simulink model "Conventional DTC"  (R2022a)
settings: Solver=ode1  StartTime=0.0  StopTime=Inf  FixedStep=Ts  RelTol=1e-3  EnableMultiTasking=on
PostLoadFcn:
  | , if any(exist('dsrtsu_mdlpostloadfcn', 'file') ~= 0), dsrtsu_mdlpostloadfcn('Execute', bdroot); end,
InitFcn:
  | , if any(exist('rtifpga_mdlclblib', 'file') ~= 0), rtifpga_mdlclblib('Init', bdroot); end,
undefined symbols (not defined in the file): P, Rs, Ts
libraries: rtilib1104 x15, rtitasklib x1
settings Model: DSRTSU_INTERNAL_RTI_VER=600  DSRTSU_INTERNAL_RTI_TYPE=rti1104  DSRTSU_INTERNAL_RTIFPGA=180  DSRTSU_INTERNAL_RTISTBM_VER=1.4.4  Creator=Admin  LastModifiedBy=acer
settings SolverCC: AlgebraicLoopSolver=TrustRegion
settings DataIOCC: LimitDataPoints=on  SaveFormat=Array  SignalLoggingSaveFormat=ModelDataLogs  ReturnWorkspaceOutputs=off
settings OptimizationCC: BlockReduction=off  ConditionallyExecuteInputs=off  OptimizeBlockIOStorage=off  BufferReuse=off  GlobalBufferReuse=off  ExpressionFolding=off  ExpressionDepthLimit=2147483647  LocalBlockOutputs=off  LifeSpan=inf
settings DebuggingCC: UnderspecifiedInitializationDetection=Classic  MergeDetectMultiDrivingBlocksExec=none  SolverPrmCheckMsg=warning  MultiTaskDSMMsg=warning  MultiTaskCondExecSysMsg=none  FcnCallInpInsideContextMsg=warning  UnconnectedInputMsg=warning  UnconnectedOutputMsg=warning  UnconnectedLineMsg=warning  StateNameClashWarn=warning  SFUnexpectedBacktrackingDiag=warning  SFNoUnconditionalDefaultTransitionDiag=warning  SFExecutionAtInitializationDiag=none  SFMachineParentedDataDiag=warning  ArithmeticOperatorsInVariantConditions=warning
settings HardwareCC: ProdBitPerPointer=32  ProdBitPerSizeT=32  ProdBitPerPtrDiffT=32  ProdLargestAtomicInteger=Integer  ProdEndianess=BigEndian  ProdWordSize=32  ProdHWDeviceType=Custom Processor->Custom  TargetIntDivRoundTo=Zero  TargetEndianess=BigEndian  TargetHWDeviceType=Custom Processor->Custom
settings ModelReferenceCC: PropagateSignalLabelsOutOfModel=off
settings SFSimCC: SimUseLocalCustomCode=off  MATLABDynamicMemAlloc=off  CustomCodeUndefinedFunction=UseInterfaceOnly
settings RTWCC: Description=dSPACE DS1104 Hardware Platform  SystemTargetFile=rti1104.tlc  MakeCommand=make_rti  TemplateMakefile=rti1104.tmf  RTWUseLocalCustomCode=off
settings CodeAppCC: StateflowObjectComments=on
settings STFCustomTargetCC: ParMdlRefBuildCompliant=on  GRTInterface=off  SystemTargetFile=rti1104.tlc
settings GRTTargetCC: TargetLangStandard=C89/C90 (ANSI)  CompOptLevelCompliant=off  ConcurrentExecutionCompliant=off  CombineOutputUpdateFcns=off  MatFileLogging=off  CPPClassGenCompliant=off  UseToolchainInfoCompliant=off  ExtModeMexFile=noextcomm
settings ConfigComp: CovMetricSettings=dw  CovSaveCumulativeToWorkspaceVar=on  CovSaveSingleToWorkspaceVar=on  CovExternalEMLEnable=off

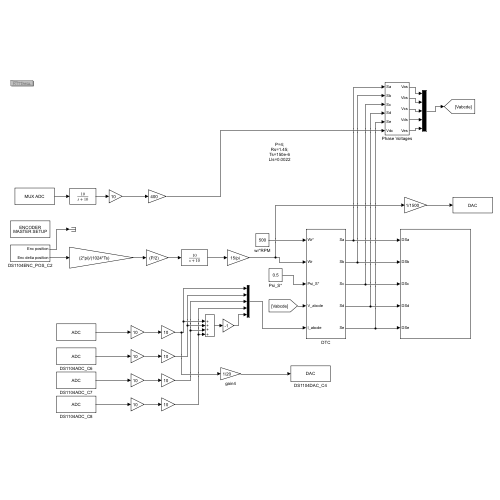
[thumbnail: Simulink's stored preview of the top-level diagram]
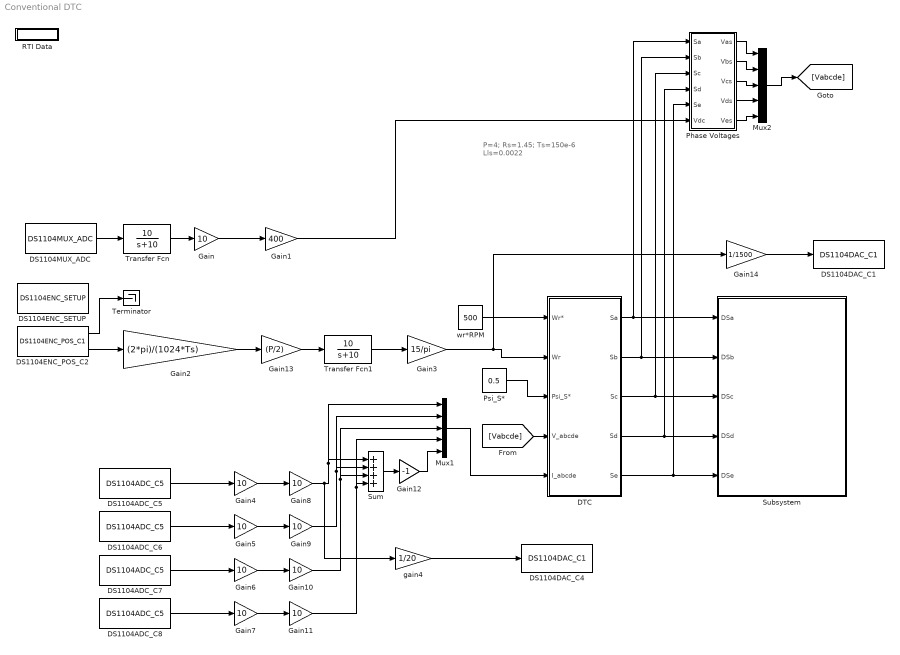
== system Conventional DTC ==
  note: P=4;
      | Rs=1.45;
      | Ts=150e-6
      | Lls=0.0022
  DS1104ADC_C5 : rtilib1104/DS1104 MASTER PPC/DS1104ADC_C5  ChannelNo=5  TriggerMode=0  Reserved1=[]  Reserved2=[]  Reserved3=[]  Reserved4=[]  DialogFcn=gui1104adc  UnitName={ 'DS1104ADC_C' }  UnitValues={ 5 }  DSProperties=struct('RTI',struct('Version',uint32(1),'BlockType',struct('isSLSource',uint8(1),'isSLSink',uint8(0),'isHWSource',uint8(1),'isHWSink',uint8(0),'isSetup',uint8(0),'isInline',uint8(1),'isNonInline',uint8(0),'isInterrupt',uint8(0),'isChannelwise',uint8(1)),'IOBoardType','DS1104MASTER','UnitType','ADC','Identifier','ADC','DialogType','ML','BlockSet','NONE','SlaveProcessor','NONE'))
      settings: SourceProductName=dSPACE RTI1104
  DS1104ADC_C6 : rtilib1104/DS1104 MASTER PPC/DS1104ADC_C5  ChannelNo=6  TriggerMode=0  Reserved1=[]  Reserved2=[]  Reserved3=[]  Reserved4=[]  DialogFcn=gui1104adc  UnitName={ 'DS1104ADC_C' }  UnitValues={ 6 }  DSProperties=struct('RTI',struct('Version',uint32(1),'BlockType',struct('isSLSource',uint8(1),'isSLSink',uint8(0),'isHWSource',uint8(1),'isHWSink',uint8(0),'isSetup',uint8(0),'isInline',uint8(1),'isNonInline',uint8(0),'isInterrupt',uint8(0),'isChannelwise',uint8(1)),'IOBoardType','DS1104MASTER','UnitType','ADC','Identifier','ADC','DialogType','ML','BlockSet','NONE','SlaveProcessor','NONE'))
      settings: SourceProductName=dSPACE RTI1104
  DS1104ADC_C7 : rtilib1104/DS1104 MASTER PPC/DS1104ADC_C5  ChannelNo=7  TriggerMode=0  Reserved1=[]  Reserved2=[]  Reserved3=[]  Reserved4=[]  DialogFcn=gui1104adc  UnitName={ 'DS1104ADC_C' }  UnitValues={ 7 }  DSProperties=struct('RTI',struct('Version',uint32(1),'BlockType',struct('isSLSource',uint8(1),'isSLSink',uint8(0),'isHWSource',uint8(1),'isHWSink',uint8(0),'isSetup',uint8(0),'isInline',uint8(1),'isNonInline',uint8(0),'isInterrupt',uint8(0),'isChannelwise',uint8(1)),'IOBoardType','DS1104MASTER','UnitType','ADC','Identifier','ADC','DialogType','ML','BlockSet','NONE','SlaveProcessor','NONE'))
      settings: SourceProductName=dSPACE RTI1104
  DS1104ADC_C8 : rtilib1104/DS1104 MASTER PPC/DS1104ADC_C5  ChannelNo=8  TriggerMode=0  Reserved1=[]  Reserved2=[]  Reserved3=[]  Reserved4=[]  DialogFcn=gui1104adc  UnitName={ 'DS1104ADC_C' }  UnitValues={ 8 }  DSProperties=struct('RTI',struct('Version',uint32(1),'BlockType',struct('isSLSource',uint8(1),'isSLSink',uint8(0),'isHWSource',uint8(1),'isHWSink',uint8(0),'isSetup',uint8(0),'isInline',uint8(1),'isNonInline',uint8(0),'isInterrupt',uint8(0),'isChannelwise',uint8(1)),'IOBoardType','DS1104MASTER','UnitType','ADC','Identifier','ADC','DialogType','ML','BlockSet','NONE','SlaveProcessor','NONE'))
      settings: SourceProductName=dSPACE RTI1104
  DS1104DAC_C1 : rtilib1104/DS1104 MASTER PPC/DS1104DAC_C1  ChannelNo=1  InitValue=0  TermMode=0  TermValue=0  Reserved1=[]  Reserved2=[]  Reserved3=[]  Reserved4=[]  DialogFcn=gui1104dac  UnitName={ 'DS1104DAC_C'}  UnitValues={ 1 }  DSProperties=struct('RTI',struct('Version',uint32(1),'BlockType',struct('isSLSource',uint8(0),'isSLSink',uint8(1),'isHWSource',uint8(0),'isHWSink',uint8(1),'isSetup',uint8(0),'isInline',uint8(1),'isNonInline',uint8(0),'isInterrupt',uint8(0),'isChannelwise',uint8(1)),'IOBoardType','DS1104MASTER','UnitType','DAC','Identifier','DAC','DialogType','ML','BlockSet','NONE','SlaveProcessor','NONE'))
      settings: SourceProductName=dSPACE RTI1104
  DS1104DAC_C4 : rtilib1104/DS1104 MASTER PPC/DS1104DAC_C1  ChannelNo=4  InitValue=0  TermMode=0  TermValue=0  Reserved1=[]  Reserved2=[]  Reserved3=[]  Reserved4=[]  DialogFcn=gui1104dac  UnitName={ 'DS1104DAC_C'}  UnitValues={4}  DSProperties=struct('RTI',struct('Version',uint32(1),'BlockType',struct('isSLSource',uint8(0),'isSLSink',uint8(1),'isHWSource',uint8(0),'isHWSink',uint8(1),'isSetup',uint8(0),'isInline',uint8(1),'isNonInline',uint8(0),'isInterrupt',uint8(0),'isChannelwise',uint8(1)),'IOBoardType','DS1104MASTER','UnitType','DAC','Identifier','DAC','DialogType','ML','BlockSet','NONE','SlaveProcessor','NONE'))
      settings: SourceProductName=dSPACE RTI1104
  DS1104ENC_POS_C2 : rtilib1104/DS1104 MASTER PPC/DS1104ENC_POS_C1  ChannelNo=2  PosValue=0  Reserved1=[]  Reserved2=[]  Reserved3=[]  Reserved4=[]  DialogFcn=gui1104enc_pos  UnitName={'DS1104ENC_POS_C'}  UnitValues={ 2 }  DSProperties=struct('RTI',struct('Version',uint32(1),'BlockType',struct('isSLSource',uint8(1),'isSLSink',uint8(0),'isHWSource',uint8(1),'isHWSink',uint8(0),'isSetup',uint8(0),'isInline',uint8(1),'isNonInline',uint8(0),'isInterrupt',uint8(0),'isChannelwise',uint8(1)),'IOBoardType','DS1104MASTER','UnitType','ENC','Identifier','ENCPOSCH','DialogType','ML','BlockSet','NONE','SlaveProcessor','NONE'))
      settings: SourceProductName=dSPACE RTI1104
  DS1104ENC_SETUP : rtilib1104/DS1104 MASTER PPC/DS1104ENC_SETUP  Reserved1=[]  Reserved2=[]  Reserved3=[]  Reserved4=[]  DialogFcn=gui1104enc_setup  UnitName={'DS1104ENC_SETUP'}  UnitValues={ [] }  DSProperties=struct('RTI',struct('Version',uint32(1),'BlockType',struct('isSLSource',uint8(0),'isSLSink',uint8(0),'isHWSource',uint8(0),'isHWSink',uint8(0),'isSetup',uint8(0),'isInline',uint8(1),'isNonInline',uint8(0),'isInterrupt',uint8(0),'isChannelwise',uint8(0)),'IOBoardType','DS1104MASTER','UnitType','ENC','Identifier','ENCSETUP','DialogType','ML','BlockSet','NONE','SlaveProcessor','NONE'))
      settings: SourceProductName=dSPACE RTI1104  SignalType=[0 0]
  DS1104MUX_ADC : rtilib1104/DS1104 MASTER PPC/DS1104MUX_ADC  ChannelNos=1  TriggerMode=0  Reserved1=[]  Reserved2=[]  Reserved3=[]  Reserved4=[]  DialogFcn=gui1104mux_adc  UnitName={ 'DS1104MUX_ADC' }  UnitValues={ [] }  DSProperties=struct('RTI',struct('Version',uint32(1),'BlockType',struct('isSLSource',uint8(1),'isSLSink',uint8(0),'isHWSource',uint8(1),'isHWSink',uint8(0),'isSetup',uint8(0),'isInline',uint8(1),'isNonInline',uint8(0),'isInterrupt',uint8(0),'isChannelwise',uint8(0)),'IOBoardType','DS1104MASTER','UnitType','ADC','Identifier','ADCMUX','DialogType','ML','BlockSet','NONE','SlaveProcessor','NONE'))
      settings: SourceProductName=dSPACE RTI1104
  DTC : Subsystem
  Gain{,4..11} (9 alike) : Gain  Gain=10
  Gain1 : Gain  Gain=400
  Gain12 : Gain  Gain=-1
  Gain13 : Gain  Gain=(P/2)
  Gain14 : Gain  Gain=1/1500
  Gain2 : Gain  Gain=(2*pi)/(1024*Ts)
  Gain3 : Gain  Gain=15/pi
  Mux1 : Mux  Inputs=5
  Mux2 : Mux  Inputs=5
  Phase Voltages : Subsystem
  Psi_S* : Constant  Value=0.5
  RTI Data : Subsystem  Tag=struct('RTIDataServer',struct('RTIDataServerVs','2','RTIModelDescription','struct(''main'',''Modified_DTC_PWMnD'',''sub'','''',''isMp'',0)'))  LoadFcn="if exist('rtidc'), try,  rtidc('DataHostBlockClbLoad', gcbh); catch, disp(['Warning: ''LoadFcn'' for RTI Data block failed: ' lasterr]); end, end,"  mask(RTI_DATA_HOST){}
      mask help:
      | RTI Data Block.
      | This block is used by RTI to store internal model-dependent data.
      | Please keep this block on the root level of the model. Deleting this block will result in data loss.
      |
      | NEVER DELETE OR COPY THIS BLOCK!
      settings: CopyFcn="if exist('rtidc'), try,  rtidc('DataHostBlockClbCopy', gcbh); catch, disp(['Warning: ''CopyFcn'' for RTI Data block failed: ' lasterr]); end, end,"  DeleteFcn="if exist('rtidc'), try,  rtidc('DataHostBlockClbDelete', gcbh); catch, disp(['Warning: ''DeleteFcn'' for RTI Data block failed: ' lasterr]); end, end,"  ModelCloseFcn="if exist('rtidc'), try,  rtidc('DataHostBlockClbModelClose', gcbh); catch, disp(['Warning: ''ModelCloseFcn'' for RTI Data block failed: ' lasterr]); end, end,"  PreSaveFcn="if exist('rtidc'), try,  rtidc('DataHostBlockClbPreSave', gcbh); catch, disp(['Warning: ''PreSaveFcn'' for RTI Data block failed: ' lasterr]); end, end,"  PostSaveFcn="if exist('rtidc'), try,  rtidc('DataHostBlockClbPostSave', gcbh); catch, disp(['Warning: ''PostSaveFcn'' for RTI Data block failed: ' lasterr]); end, end,"  NameChangeFcn="if exist('rtidc'), try,  rtidc('DataHostBlockClbNameChange', gcbh); catch, disp(['Warning: ''NameChangeFcn'' for RTI Data block failed: ' lasterr]); end, end,"
      mask Help:
      | RTI Data Block.
      | This block is used by RTI to store internal model-dependent data.
      | Please keep this block on the root level of the model. Deleting this block will result in data loss.
      | 
      | NEVER DELETE OR COPY THIS BLOCK!
      mask Display:
      | text(0.5, 0.5, 'RTI Data', 'HorizontalAlignment', 'center');
      | plot([1 0]);
  Subsystem : Subsystem
  Sum : Sum  Inputs=|++++
  Terminator : Terminator
  Transfer Fcn : TransferFcn  Numerator=[10]  Denominator=[1 10]
  Transfer Fcn1 : TransferFcn  Numerator=[10]  Denominator=[1 10]
  gain4 : Gain  Gain=1/20  SaturateOnIntegerOverflow=on  OutDataTypeStr=Inherit: Same as input  ParamDataTypeStr=Inherit: Same as input
  wr*RPM : Constant  Value=500
  wires:
  wr*RPM/1 -> DTC/1(Wr*)
  [Vabcde] -> DTC/4(V_abcde)
  Psi_S*/1 -> DTC/3(Psi_S*)
  Gain/1 -> Gain1/1
  Transfer Fcn/1 -> Gain/1
  Gain4/1 -> Gain8/1
  Gain5/1 -> Gain9/1
  Gain6/1 -> Gain10/1
  Gain7/1 -> Gain11/1
  Gain9/1 -> Mux1/2, Sum/2
  Gain10/1 -> Mux1/3, Sum/3
  Gain11/1 -> Mux1/4, Sum/4
  Mux1/1 -> DTC/5(I_abcde)
  Phase Voltages/1(Vas) -> Mux2/1
  Phase Voltages/2(Vbs) -> Mux2/2
  Phase Voltages/3(Vcs) -> Mux2/3
  Phase Voltages/4(Vds) -> Mux2/4
  Phase Voltages/5(Ves) -> Mux2/5
  Mux2/1 -> [Vabcde]
  DTC/1(Sa) -> Phase Voltages/1(Sa), Subsystem/1(DSa)
  DTC/2(Sb) -> Subsystem/2(DSb), Phase Voltages/2(Sb)
  DTC/3(Sc) -> Subsystem/3(DSc), Phase Voltages/3(Sc)
  DTC/4(Sd) -> Subsystem/4(DSd), Phase Voltages/4(Sd)
  DTC/5(Se) -> Subsystem/5(DSe), Phase Voltages/5(Se)
  Sum/1 -> Gain12/1
  Gain12/1 -> Mux1/5
  DS1104ADC_C5/1 -> Gain4/1
  DS1104ADC_C6/1 -> Gain5/1
  DS1104ADC_C7/1 -> Gain6/1
  DS1104ADC_C8/1 -> Gain7/1
  Transfer Fcn1/1 -> Gain3/1
  DS1104MUX_ADC/1 -> Transfer Fcn/1
  DS1104ENC_POS_C2/2 -> Gain2/1
  Gain2/1 -> Gain13/1
  Gain13/1 -> Transfer Fcn1/1
  DS1104ENC_POS_C2/1 -> Terminator/1
  Gain1/1 -> Phase Voltages/6(Vdc)
  Gain14/1 -> DS1104DAC_C1/1
  Gain3/1 -> Gain14/1, DTC/2(Wr)
  Gain8/1 -> gain4/1, Mux1/1, Sum/1
  gain4/1 -> DS1104DAC_C4/1

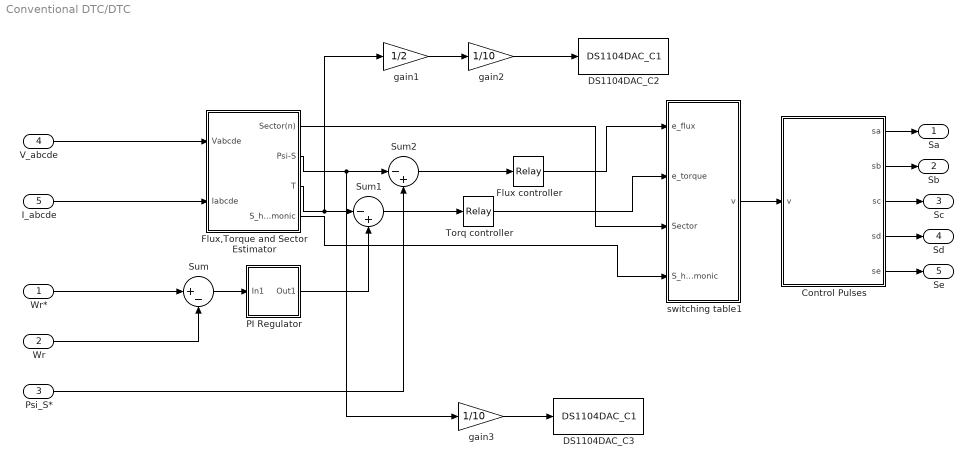
== system Conventional DTC/DTC ==
  Wr* : Inport
  Wr : Inport  Port=2
  Psi_S* : Inport  Port=3
  V_abcde : Inport  Port=4
  I_abcde : Inport  Port=5
  Control Pulses : MATLAB Function  TreatAsAtomicUnit=on
  DS1104DAC_C2 : rtilib1104/DS1104 MASTER PPC/DS1104DAC_C1  ChannelNo=2  InitValue=0  TermMode=0  TermValue=0  Reserved1=[]  Reserved2=[]  Reserved3=[]  Reserved4=[]  DialogFcn=gui1104dac  UnitName={ 'DS1104DAC_C'}  UnitValues={ 2 }  DSProperties=struct('RTI',struct('Version',uint32(1),'BlockType',struct('isSLSource',uint8(0),'isSLSink',uint8(1),'isHWSource',uint8(0),'isHWSink',uint8(1),'isSetup',uint8(0),'isInline',uint8(1),'isNonInline',uint8(0),'isInterrupt',uint8(0),'isChannelwise',uint8(1)),'IOBoardType','DS1104MASTER','UnitType','DAC','Identifier','DAC','DialogType','ML','BlockSet','NONE','SlaveProcessor','NONE'))
      settings: SourceProductName=dSPACE RTI1104
  DS1104DAC_C3 : rtilib1104/DS1104 MASTER PPC/DS1104DAC_C1  ChannelNo=3  InitValue=0  TermMode=0  TermValue=0  Reserved1=[]  Reserved2=[]  Reserved3=[]  Reserved4=[]  DialogFcn=gui1104dac  UnitName={ 'DS1104DAC_C'}  UnitValues={ 3 }  DSProperties=struct('RTI',struct('Version',uint32(1),'BlockType',struct('isSLSource',uint8(0),'isSLSink',uint8(1),'isHWSource',uint8(0),'isHWSink',uint8(1),'isSetup',uint8(0),'isInline',uint8(1),'isNonInline',uint8(0),'isInterrupt',uint8(0),'isChannelwise',uint8(1)),'IOBoardType','DS1104MASTER','UnitType','DAC','Identifier','DAC','DialogType','ML','BlockSet','NONE','SlaveProcessor','NONE'))
      settings: SourceProductName=dSPACE RTI1104
  Flux controller : Relay  OnSwitchValue=0.01  OffSwitchValue=-0.01  OffOutputValue=-1
  Flux,Torque and Sector Estimator : Subsystem
  PI Regulator : Subsystem
  Sum : Sum  Inputs=|+-
  Sum1 : Sum  Inputs=|-+
  Sum2 : Sum  Inputs=|-+
  Torq controller : Relay  OnSwitchValue=0.5  OffSwitchValue=-0.5  OffOutputValue=-1
  gain1 : Gain  Gain=1/2  SaturateOnIntegerOverflow=on  OutDataTypeStr=Inherit: Same as input  ParamDataTypeStr=Inherit: Same as input
  gain2 : Gain  Gain=1/10  SaturateOnIntegerOverflow=on  OutDataTypeStr=Inherit: Same as input  ParamDataTypeStr=Inherit: Same as input
  gain3 : Gain  Gain=1/10  SaturateOnIntegerOverflow=on  OutDataTypeStr=Inherit: Same as input  ParamDataTypeStr=Inherit: Same as input
  switching table1 : Subsystem
  Sa : Outport
  Sb : Outport  Port=2
  Sc : Outport  Port=3
  Sd : Outport  Port=4
  Se : Outport  Port=5
  wires:
  PI Regulator/1(Out1) -> Sum1/2
  Flux controller/1 -> switching table1/1(e_flux)
  Sum2/1 -> Flux controller/1
  Wr/1 -> Sum/2
  Psi_S*/1 -> Sum2/2
  Sum/1 -> PI Regulator/1(In1)
  V_abcde/1 -> Flux,Torque and Sector Estimator/1(Vabcde)
  switching table1/1(v) -> Control Pulses/1(v)
  Control Pulses/1(sa) -> Sa/1
  Control Pulses/2(sb) -> Sb/1
  Control Pulses/3(sc) -> Sc/1
  Control Pulses/4(sd) -> Sd/1
  Control Pulses/5(se) -> Se/1
  I_abcde/1 -> Flux,Torque and Sector Estimator/2(Iabcde)
  Sum1/1 -> Torq controller/1
  Torq controller/1 -> switching table1/2(e_torque)
  Flux,Torque and Sector Estimator/4(S_harmonic) -> switching table1/4(S_harmonic)
  Wr*/1 -> Sum/1
  gain1/1 -> gain2/1
  gain2/1 -> DS1104DAC_C2/1
  Flux,Torque and Sector Estimator/3(T) -> gain1/1, Sum1/1
  gain3/1 -> DS1104DAC_C3/1
  Flux,Torque and Sector Estimator/2(Psi-S) -> gain3/1, Sum2/1
  Flux,Torque and Sector Estimator/1(Sector(n)) -> switching table1/3(Sector)

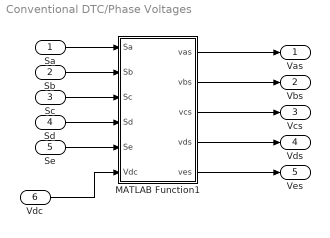
== system Conventional DTC/Phase Voltages ==
  Sa : Inport
  Sb : Inport  Port=2
  Sc : Inport  Port=3
  Sd : Inport  Port=4
  Se : Inport  Port=5
  Vdc : Inport  Port=6
  MATLAB Function1 : MATLAB Function  TreatAsAtomicUnit=on
  Vas : Outport
  Vbs : Outport  Port=2
  Vcs : Outport  Port=3
  Vds : Outport  Port=4
  Ves : Outport  Port=5
  wires:
  Sa/1 -> MATLAB Function1/1(Sa)
  Sb/1 -> MATLAB Function1/2(Sb)
  Sc/1 -> MATLAB Function1/3(Sc)
  Sd/1 -> MATLAB Function1/4(Sd)
  Se/1 -> MATLAB Function1/5(Se)
  MATLAB Function1/1(vas) -> Vas/1
  MATLAB Function1/4(vds) -> Vds/1
  MATLAB Function1/5(ves) -> Ves/1
  Vdc/1 -> MATLAB Function1/6(Vdc)
  MATLAB Function1/2(vbs) -> Vbs/1
  MATLAB Function1/3(vcs) -> Vcs/1

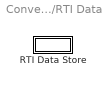
== system Conventional DTC/RTI Data ==
  RTI Data Store : Subsystem  Tag="struct('public',struct('sub',struct('name',{{'Modified_DTC_PWMnD'}},'data',{{struct('TH',struct('thTaskInfo',struct('taskType',{'TIMER','HWINT','TMRINT','SWINT','GLINT'},'tasksNumOf',{1,0,0,0,0},'srcIds',{{'PWMINT'},{},{},{},{}},'taskNames',{{['Timer Task 1']},{},{},{},{}})),'th_tc',struct('dataType','TASK','taskGroupId','','taskGroupList',{{}},'taskSchedulingPolicy','FCFS','taskType','TIMER','blkh','Modified_DTC_PWMnD/Subsystem/DS1104SLAVE_PWMINT1','srcId','PWMINT','srcSgnName',['SLAVE-PWM-Interrupt with variable alignment'],'srcCpuName','','taskName',['Timer Task 1  [0.00015] s'],'taskNameDisplayExt','','smplTime',0.00015,'smplTimeOffs',0,'hasFixedPriority',0,'priority',1,'hasFixedOvc',0,'ovcType',1,'ovcMax',1),'tc_th',struct('dataType','TASK','taskGroupId','','taskGroupList',{{}},'taskSchedulingPolicy','FCFS','taskType','TIMER','blkh','Modified_DTC_PWMnD/Subsystem/DS1104SLAVE_PWMINT1','srcId','PWMINT','srcSgnName',['SLAVE-PWM-Interrupt with variable alignment'],'srcCpuName','','taskName',['Timer Task 1  [0.00015] s'],'taskNameDisplayExt','','smplTime',0.00015,'smplTimeOffs',0,'hasFixedPriority',0,'priority',1,'hasFixedOvc',0,'ovcType',1,'ovcMax',1))}})),'private',struct('version',struct('dsVer',uint32(2)),'access',struct('modified',['16-Jul-2024 11:25:11'],'type','Model','isPerm',1)))"  mask(RTI_DATA_STORE){}
      mask help:
      | RTI Data Store Block. This block is used by RTI to store internal model dependent data. Deleting this block will result in data loss.
      |
      | NEVER DELETE, COPY, OR MODIFY THIS BLOCK!
      mask Help:
      | RTI Data Store Block. This block is used by RTI to store internal model dependent data. Deleting this block will result in data loss.
      | 
      | NEVER DELETE, COPY, OR MODIFY THIS BLOCK!
      mask Display: text(0.5, 0.5, ' ', 'HorizontalAlignment', 'center');

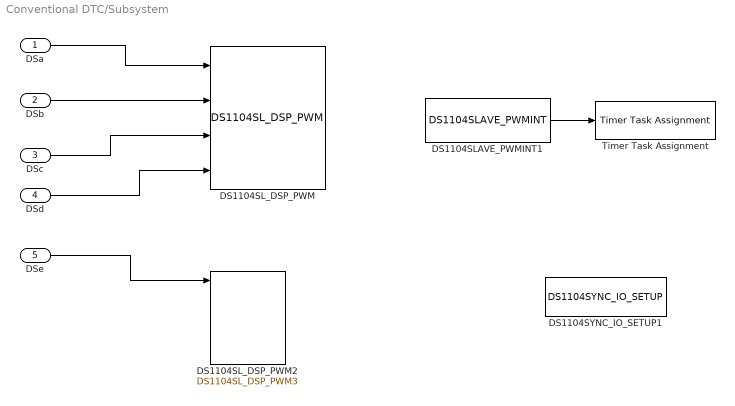
== system Conventional DTC/Subsystem ==
  DSa : Inport
  DSb : Inport  Port=2
  DSc : Inport  Port=3
  DSd : Inport  Port=4
  DSe : Inport  Port=5
  DS1104SLAVE_PWMINT1 : rtilib1104/DS1104 SLAVE DSP/DS1104SLAVE_PWMINT  Parameters=[]  TDef=[]  BoardIntNo=[]  InterruptName=[]  Delay=[]  DialogFcn=[]  Reserved1=[]  Reserved2=[]  Reserved3=[]  Reserved4=[]  Revision=[]  UnitName=[]  UnitValues=[]  DSProperties=struct('RTI',struct('Version',uint32(530),'IOBoardType','DS1104SLAVE','SlaveProcessor','F240','UnitType','HWINT','Identifier','PWMINT','BlockType',struct('isSLSource',uint8(1),'isSLSink',uint8(0),'isHWSource',uint8(1),'isHWSink',uint8(0),'isSetup',uint8(0),'isInline',uint8(1),'isNonInline',uint8(0),'isInterrupt',uint8(1),'isChannelwise',uint8(0)),'DialogType','ML','BlockSet','NONE','RelationId',struct('TH',struct('BlockId','HWINT'))))  RTIBlockInterface=struct('BlockName',struct('Token',{{'DS1104SLAVE_PWMINT'}}),'BlockDisplay',{{['DS1104SLAVE Board \nPWM-Interrupt'],'center'}},'DialogFcn','rti110xhwintgui','OutputPortsActive',1,'OutputPortsWidth',int32(1),'FunctionCall',uint32(0),'OutputPortsName',{{[' ']}},'IconTransparency','on','InitLevel',3,'Options',{{'SS_OPTION_FORCE_NONINLINED_FCNCALL','SS_OPTION_ASYNCHRONOUS_INTERRUPT'}},'OutputPortsDataType',{{'SS_FCN_CALL'}})  RTIBlockParameters=struct('ThIntNo',{{10,'OFF',[]}},'IntDelay',{{0.01,'ON',[1e-6 1]}},'ThSrcSgnName',{{['SLAVE-PWM-Interrupt with variable alignment'],'OFF',[]}},'TLCFileName',{{'rti1104slave_pwm_interrupt','OFF',[]}},'ThBlk',{{['struct(''blkh'',''Modified_DTC_PWMnD/Subsystem/DS1104SLAVE_PWMINT1'',''srcId'',''PWMINT'',''srcSgnId'',''PWMINT'',''intervalTmrBlockId'',[],''srcSgnName'',[''SLAVE-PWM-Interrupt with variable alignment''],''srcCpuId'','''',''isSrcCpu'',1,''isTargetCpu'',1,''srcOnMasterCpu'',1,''boardType'','''',''boardTypeNo'','''',''boardNo'',1,''intNo'',0,''subIntNo'',-1,''period'',0,''entryPoint'',''rti_PWMINT'',''blockName'',''DS1104SLAVE_PWMINT1'',''taskNameDisplayExt'','''',''taskType'',''HWINT'',''groupId'',''PWMINT'',''hookFcn'',''NULL'',''isTimerTaskSrc'',1,''service'','''',''mpBlkId'','''',''taskPriorityPreConfig'',''none'',''taskPriority'',-1,''taskSortWeighting'',[],''taskSchedulingPolicy'',''FCFS'',''taskOvrPreConfig'',''none'',''taskOvrStrategy'',1,''taskOvrQueueSize'',1,''taskVisibility'',''on'',''taskGroupId'','''',''taskGroupDisplayOrder'',[],''serviceDynamicGen'',0,''disableCodeGen'',0,''boardBase'',''0'',''noBoardBase'','''')'],'OFF',[]}},'PHSBoardBaseId',{{'DSXXXX','OFF',[]}})  RTISFcnParameters=struct('IntDelay','double','ThBlk','struct','ThIntNo','int32','TLCFileName','char','PHSBoardBaseId','char')  RTIBlockParaDefault=struct('ThIntNo',10,'IntDelay',2^-1,'ThSrcSgnName',['SLAVE-PWM-Interrupt with none delay'],'TLCFileName','rti1104slave_pwm_interrupt','ThBlk',['struct(''srcSgnId'', '''')'],'PHSBoardBaseId','DSXXXX')
      settings: SourceProductName=dSPACE RTI1104
  DS1104SL_DSP_PWM : rtilib1104/DS1104 SLAVE DSP/DS1104SL_DSP_PWM  Parameters=[]  TDef=[]  BoardType=[]  PwmMode=[]  Frequency=[]  InitValue=[]  TermMode=[]  TermValue=[]  Polarity=[]  DialogFcn=[]  Reserved1=[]  Reserved2=[]  Reserved3=[]  Reserved4=[]  Revision=[]  UnitName=[]  UnitValues=[]  DSProperties=struct('RTI',struct('Version',uint32(2),'BlockType',struct('isSLSource',uint8(0),'isSLSink',uint8(1),'isHWSource',uint8(0),'isHWSink',uint8(1),'isSetup',uint8(0),'isInline',uint8(1),'isNonInline',uint8(0),'isInterrupt',uint8(0),'isChannelwise',uint8(0)),'IOBoardType','DS1104SLAVE','UnitType','PWM','Identifier','PWM','DialogType','ML','BlockSet','NONE','SlaveProcessor','F240'))  RTIBlockInterface=struct('InputPortsActive',[1 1 1 1],'InputPortsWidth',int32([1 1 1 1]),'InputPortsName',{{['PWM Channel 1'],['PWM Channel 2'],['PWM Channel 3'],['PWM Channel 4']}},'IWork',{{{'',uint32(4)}}},'DialogFcn','rti1104slavepwmgui','InitLevel',1,'BlockDisplay',{{'','auto'}},'IconTransparency','on','MultiSFcn',4,'BlockName',struct('Token',{{'DS1104SL_DSP_PWM'}}))  RTIBlockParameters=struct('PWMSymmetryMode',{{1,'OFF',[]}},'PWMFrequency',{{'1/Ts','OFF',[]}},'PWMPolarityMode',{{[1 1 1 1 1],'OFF',[]}},'ChannelNo',{{[1 2 3 4],'OFF',[]}},'SuspendModeInit',{{[1 1 1 1 1],'OFF',[]}},'TTLModeInit',{{[2 2 2 2 2],'OFF',[]}},'DutyCycleInitValueCh1',{{'0.5','OFF',[]}},'DutyCycleInitValueCh2',{{'0.5','OFF',[]}},'DutyCycleInitValueCh3',{{'0.5','OFF',[]}},'DutyCycleInitValueCh4',{{'0.5','OFF',[]}},'DutyCycleInitValueCh5',{{'0.5','OFF',[]}},'EnablePWMStop',{{[0 0 0 0 0],'OFF',[]}},'SuspendModeTerm',{{[0 1 1 1 1],'OFF',[]}},'TTLModeTerm',{{[2 2 2 2 2],'OFF',[]}},'DutyCycleTermValueCh1',{{'0.5','OFF',[]}},'DutyCycleTermValueCh2',{{'0.5','OFF',[]}},'DutyCycleTermValueCh3',{{'0.5','OFF',[]}},'DutyCycleTermValueCh4',{{'0.5','OFF',[]}},'DutyCycleTermValueCh5',{{'0.5','OFF',[]}},'TLCFileName',{{'rti1104pwm','OFF',[]}})  RTISFcnParameters=struct('PWMSymmetryMode','double','PWMFrequency','double','PWMPolarityMode','double','ChannelNo','double','SuspendModeInit','double','TTLModeInit','double','DutyCycleInitValueCh1','double','DutyCycleInitValueCh2','double','DutyCycleInitValueCh3','double','DutyCycleInitValueCh4','double','EnablePWMStop','double','SuspendModeTerm','double','TTLModeTerm','double','DutyCycleTermValueCh1','double','DutyCycleTermValueCh2','double','DutyCycleTermValueCh3','double','DutyCycleTermValueCh4','double','TLCFileName','char')  RTIBlockParaDefault=struct('PWMSymmetryMode',1,'PWMFrequency',100,'PWMPolarityMode',[1 1 1 1 1],'ChannelNo',[1 2 3 4],'SuspendModeInit',[1 1 1 1 1],'TTLModeInit',[2 2 2 2 2],'DutyCycleInitValueCh1',2^-1,'DutyCycleInitValueCh2',2^-1,'DutyCycleInitValueCh3',2^-1,'DutyCycleInitValueCh4',2^-1,'DutyCycleInitValueCh5',2^-1,'EnablePWMStop',[1 1 1 1 0],'SuspendModeTerm',[1 1 1 1 1],'TTLModeTerm',[2 2 2 2 2],'DutyCycleTermValueCh1',2^-1,'DutyCycleTermValueCh2',2^-1,'DutyCycleTermValueCh3',2^-1,'DutyCycleTermValueCh4',2^-1,'DutyCycleTermValueCh5',2^-1,'TLCFileName','rti1104pwm')
      settings: SourceProductName=dSPACE RTI1104
  DS1104SL_DSP_PWM2 : rtilib1104/DS1104 SLAVE DSP/DS1104SL_DSP_PWM3  Parameters=[]  TDef=[]  BoardType=[]  PwmMode=[]  Frequency=[]  DeadBand=[]  InitValue=[]  TermMode=[]  TermValue=[]  IntDelay=[]  DialogFcn=[]  Reserved1=[]  Reserved2=[]  Reserved3=[]  Reserved4=[]  Revision=[]  UnitName=[]  UnitValues=[]  DSProperties=struct('RTI',struct('Version',uint32(2),'BlockType',struct('isSLSource',uint8(0),'isSLSink',uint8(1),'isHWSource',uint8(0),'isHWSink',uint8(1),'isSetup',uint8(0),'isInline',uint8(1),'isNonInline',uint8(0),'isInterrupt',uint8(0),'isChannelwise',uint8(0)),'IOBoardType','DS1104SLAVE','UnitType','PWM','Identifier','PWM3','DialogType','ML','BlockSet','NONE','SlaveProcessor','F240'))  RTIBlockInterface=struct('InputPortsActive',[1 1 1 1],'InputPortsWidth',int32([1 1 1 1]),'InputPortsName',{{['Duty cycle a'],['Duty cycle b'],['Duty cycle c'],['PWM Stop']}},'IWork',{{{'',uint32(1)}}},'DialogFcn','rti1104slavepwm3gui','InitLevel',1,'BlockDisplay',{{'','auto'}},'IconTransparency','on','BlockName',struct('Token',{{'DS1104SL_DSP_PWM3'}}))  RTIBlockParameters=struct('PWMFrequency',{{'1/Ts','OFF',[]}},'PWMDeadband',{{'0','OFF',[]}},'PWMPolarityMode',{{[1 1 1 1],'OFF',[]}},'PWMPolarityInvMode',{{[2 2 2 2],'OFF',[]}},'SuspendModeInit',{{[1 1 1],'OFF',[]}},'TTLModeInit',{{[2 2 2],'OFF',[]}},'TTLModeInitNOT',{{[1 1 1],'OFF',[]}},'DutyCycleInitValueCh1',{{'0.5','OFF',[]}},'DutyCycleInitValueCh2',{{'0.5','OFF',[]}},'DutyCycleInitValueCh3',{{'0.5','OFF',[]}},'EnablePWMStop',{{1,'OFF',[]}},'SuspendModeTerm',{{[1 1 1],'OFF',[]}},'TTLModeTerm',{{[2 2 2],'OFF',[]}},'TTLModeTermNOT',{{[1 1 1],'OFF',[]}},'DutyCycleTermValueCh1',{{'0.5','OFF',[]}},'DutyCycleTermValueCh2',{{'0.5','OFF',[]}},'DutyCycleTermValueCh3',{{'0.5','OFF',[]}},'TLCFileName',{{'rti1104pwm3','OFF',[]}})  RTISFcnParameters=struct('PWMFrequency','double','PWMDeadband','double','PWMPolarityMode','double','PWMPolarityInvMode','double','SuspendModeInit','double','TTLModeInit','double','TTLModeInitNOT','double','DutyCycleInitValueCh1','double','DutyCycleInitValueCh2','double','DutyCycleInitValueCh3','double','EnablePWMStop','double','SuspendModeTerm','double','TTLModeTerm','double','TTLModeTermNOT','double','DutyCycleTermValueCh1','double','DutyCycleTermValueCh2','double','DutyCycleTermValueCh3','double','TLCFileName','char')  RTIBlockParaDefault=struct('PWMFrequency',100,'PWMDeadband',50,'PWMPolarityMode',[1 1 1 1],'PWMPolarityInvMode',[2 2 2 2],'SuspendModeInit',[1 1 1],'TTLModeInit',[2 2 2],'TTLModeInitNOT',[1 1 1],'DutyCycleInitValueCh1',2^-1,'DutyCycleInitValueCh2',2^-1,'DutyCycleInitValueCh3',2^-1,'EnablePWMStop',1,'SuspendModeTerm',[1 1 1],'TTLModeTerm',[2 2 2],'TTLModeTermNOT',[1 1 1],'DutyCycleTermValueCh1',2^-1,'DutyCycleTermValueCh2',2^-1,'DutyCycleTermValueCh3',2^-1,'TLCFileName','rti1104pwm3')
      settings: SourceProductName=dSPACE RTI1104
  DS1104SYNC_IO_SETUP1 : rtilib1104/DS1104 MASTER PPC/DS1104SYNC_IO_SETUP  DSProperties=struct('RTI',struct('Version',uint32(1),'BlockType',struct('isSLSource',uint8(0),'isSLSink',uint8(0),'isHWSource',uint8(0),'isHWSink',uint8(0),'isSetup',uint8(1),'isInline',uint8(1),'isNonInline',uint8(0),'isInterrupt',uint8(0),'isChannelwise',uint8(0)),'IOBoardType','DS1104MASTER','UnitType','SETUP','Identifier','SYNCSETUP','DialogType','ML','BlockSet','NONE','SlaveProcessor','NONE'))  RTIBlockInterface=struct('OutputPortsActive',0,'OutputPortsWidth',int32(0),'DialogFcn','gui1104mastersyncsetup','InitLevel',1,'BlockDisplay',{{['Master Sync IO Setup'],'center'}},'IconTransparency','off','BlockName',struct('Token',{{'DS1104SYNC_IO_SETUP'}}))  RTIBlockParameters=struct('TriggerSource',{{1,'OFF',[]}},'SyncIn',{{2,'OFF',[]}},'SyncOut',{{2,'OFF',[]}},'SyncADC',{{[0 0 0 0 0],'OFF',[]}},'SyncDAC',{{0,'OFF',[]}},'SyncInc',{{[0 0],'OFF',[]}},'TLCFileName',{{'rti1104mastersyncsetup','OFF',[]}})  RTISFcnParameters=struct('TriggerSource','int32','SyncIn','int32','SyncOut','int32','SyncADC','int32','SyncDAC','int32','SyncInc','int32','TLCFileName','char')  RTIBlockParaDefault=struct('TriggerSource',1,'SyncIn',1,'SyncOut',1,'SyncADC',[0 0 0 0 0],'SyncDAC',0,'SyncInc',[0 0],'TLCFileName','rti1104mastersyncsetup')
      settings: SourceProductName=dSPACE RTI1104
  Timer Task Assignment : rtitasklib/Timer Task Assignment  Reserved2=[]  Reserved3=[]  Reserved4=[]  DSProperties=struct('RTI',struct('Version',uint32(2),'BlockType',struct('isSLSource',uint8(0),'isSLSink',uint8(1),'isHWSource',uint8(0),'isHWSink',uint8(0),'isSetup',uint8(0),'isInline',uint8(1),'isNonInline',uint8(0),'isInterrupt',uint8(0),'isChannelwise',uint8(0)),'IOBoardType','INTLIB','UnitType','TTASSIGN','Identifier','TTASSIGN','DialogType','SL','BlockSet','NONE','SlaveProcessor','NONE','RelationId',struct('TH',struct('BlockId','TTASSIGN'))))
  wires:
  DSc/1 -> DS1104SL_DSP_PWM/3
  DSe/1 -> DS1104SL_DSP_PWM2/1
  DSa/1 -> DS1104SL_DSP_PWM/1
  DSb/1 -> DS1104SL_DSP_PWM/2
  DSd/1 -> DS1104SL_DSP_PWM/4
  DS1104SLAVE_PWMINT1/1 -> Timer Task Assignment/1

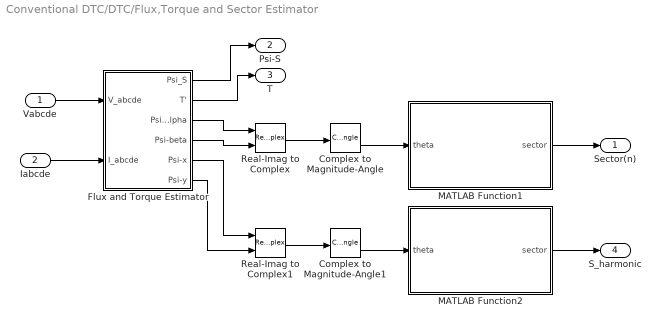
== system Conventional DTC/DTC/Flux,Torque and Sector Estimator ==
  Vabcde : Inport
  Iabcde : Inport  Port=2
  Complex to Magnitude-Angle : ComplexToMagnitudeAngle
  Complex to Magnitude-Angle1 : ComplexToMagnitudeAngle
  Flux and Torque Estimator : Subsystem
  MATLAB Function1 : MATLAB Function  TreatAsAtomicUnit=on
  MATLAB Function2 : MATLAB Function  TreatAsAtomicUnit=on
  Real-Imag to Complex : RealImagToComplex
  Real-Imag to Complex1 : RealImagToComplex
  Sector(n) : Outport
  Psi-S : Outport  Port=2
  T : Outport  Port=3
  S_harmonic : Outport  Port=4
  wires:
  Flux and Torque Estimator/2(T') -> T/1
  Flux and Torque Estimator/1(Psi_S) -> Psi-S/1
  MATLAB Function1/1(sector) -> Sector(n)/1
  Vabcde/1 -> Flux and Torque Estimator/1(V_abcde)
  Iabcde/1 -> Flux and Torque Estimator/2(I_abcde)
  Flux and Torque Estimator/3(Psi-alpha) -> Real-Imag to Complex/1
  Flux and Torque Estimator/4(Psi-beta) -> Real-Imag to Complex/2
  Real-Imag to Complex/1 -> Complex to Magnitude-Angle/1
  Complex to Magnitude-Angle/2 -> MATLAB Function1/1(theta)
  Flux and Torque Estimator/5(Psi-x) -> Real-Imag to Complex1/1
  Flux and Torque Estimator/6(Psi-y) -> Real-Imag to Complex1/2
  Real-Imag to Complex1/1 -> Complex to Magnitude-Angle1/1
  Complex to Magnitude-Angle1/2 -> MATLAB Function2/1(theta)
  MATLAB Function2/1(sector) -> S_harmonic/1

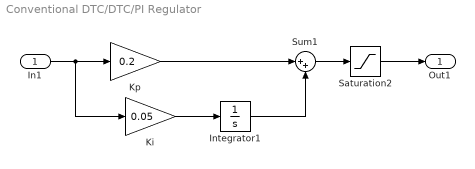
== system Conventional DTC/DTC/PI Regulator ==
  In1 : Inport
  Integrator1 : Integrator  LimitOutput=on  UpperSaturationLimit=14  LowerSaturationLimit=-14
  Ki : Gain  Gain=0.05
  Kp : Gain  Gain=0.2
  Saturation2 : Saturate  UpperLimit=14  LowerLimit=-14
  Sum1 : Sum  Inputs=|++
  Out1 : Outport
  wires:
  Ki/1 -> Integrator1/1
  Kp/1 -> Sum1/1
  Integrator1/1 -> Sum1/2
  Sum1/1 -> Saturation2/1
  In1/1 -> Kp/1, Ki/1
  Saturation2/1 -> Out1/1

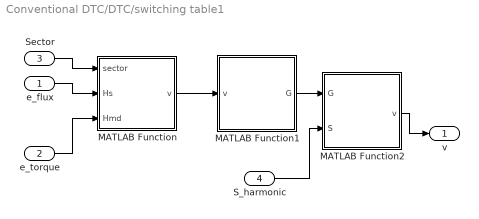
== system Conventional DTC/DTC/switching table1 ==
  e_flux : Inport
  e_torque : Inport  Port=2
  Sector : Inport  Port=3
  S_harmonic : Inport  Port=4
  MATLAB Function : MATLAB Function  TreatAsAtomicUnit=on
  MATLAB Function1 : MATLAB Function  TreatAsAtomicUnit=on
  MATLAB Function2 : MATLAB Function  TreatAsAtomicUnit=on
  v : Outport
  wires:
  MATLAB Function2/1(v) -> v/1
  S_harmonic/1 -> MATLAB Function2/2(S)
  MATLAB Function/1(v) -> MATLAB Function1/1(v)
  MATLAB Function1/1(G) -> MATLAB Function2/1(G)
  Sector/1 -> MATLAB Function/1(sector)
  e_flux/1 -> MATLAB Function/2(Hs)
  e_torque/1 -> MATLAB Function/3(Hmd)

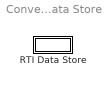
== system Conventional DTC/RTI Data/RTI Data Store ==
  RTI Data Store : Subsystem  mask(RTI_DATA_STORE){}
      mask help:
      | RTI Data Store Block. This block is used by RTI to store internal model dependent data. Deleting this block will result in data loss.
      |
      | NEVER DELETE, COPY, OR MODIFY THIS BLOCK!
      mask Help:
      | RTI Data Store Block. This block is used by RTI to store internal model dependent data. Deleting this block will result in data loss.
      | 
      | NEVER DELETE, COPY, OR MODIFY THIS BLOCK!
      mask Display: text(0.5, 0.5, ' ', 'HorizontalAlignment', 'center');

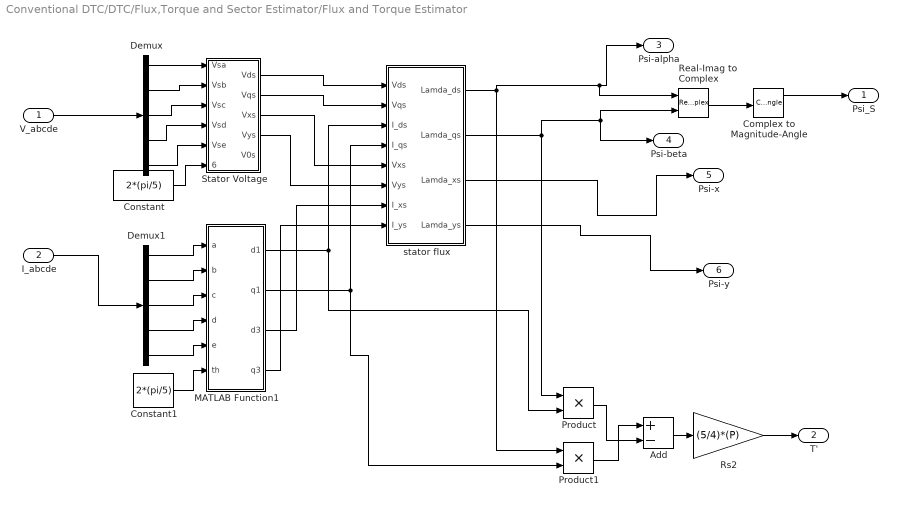
== system Conventional DTC/DTC/Flux,Torque and Sector Estimator/Flux and Torque Estimator ==
  V_abcde : Inport
  I_abcde : Inport  Port=2
  Add : Sum  Inputs=+-
  Complex to Magnitude-Angle : ComplexToMagnitudeAngle
  Constant : Constant  Value=2*(pi/5)
  Constant1 : Constant  Value=2*(pi/5)
  Demux : Demux  Outputs=5
  Demux1 : Demux  Outputs=5
  MATLAB Function1 : MATLAB Function  TreatAsAtomicUnit=on
  Product : Product
  Product1 : Product
  Real-Imag to Complex : RealImagToComplex
  Rs2 : Gain  Gain=(5/4)*(P)
  "Stator Voltage " : Subsystem
  stator flux : Subsystem
  Psi_S : Outport
  T' : Outport  Port=2
  Psi-alpha : Outport  Port=3
  Psi-beta : Outport  Port=4
  Psi-x : Outport  Port=5
  Psi-y : Outport  Port=6
  wires:
  I_abcde/1 -> Demux1/1
  Demux1/1 -> MATLAB Function1/1(a)
  Demux1/3 -> MATLAB Function1/3(c)
  Demux1/2 -> MATLAB Function1/2(b)
  V_abcde/1 -> Demux/1
  Add/1 -> Rs2/1
  Complex to Magnitude-Angle/1 -> Psi_S/1
  Rs2/1 -> T'/1
  Demux/1 -> "Stator Voltage "/1(Vsa)
  Demux/2 -> "Stator Voltage "/2(Vsb)
  Demux/3 -> "Stator Voltage "/3(Vsc)
  Demux/4 -> "Stator Voltage "/4(Vsd)
  Demux/5 -> "Stator Voltage "/5(Vse)
  Demux1/4 -> MATLAB Function1/4(d)
  Demux1/5 -> MATLAB Function1/5(e)
  Constant/1 -> "Stator Voltage "/6(2*pi/5)
  "Stator Voltage "/2(Vqs) -> stator flux/2(Vqs)
  "Stator Voltage "/1(Vds) -> stator flux/1(Vds)
  MATLAB Function1/2(q1) -> Product1/2, stator flux/4(I_qs)
  "Stator Voltage "/3(Vxs) -> stator flux/5(Vxs)
  "Stator Voltage "/4(Vys) -> stator flux/6(Vys)
  stator flux/3(Lamda_xs) -> Psi-x/1
  stator flux/4(Lamda_ys) -> Psi-y/1
  Constant1/1 -> MATLAB Function1/6(th)
  MATLAB Function1/1(d1) -> Product/2, stator flux/3(I_ds)
  Product1/1 -> Add/1
  Product/1 -> Add/2
  MATLAB Function1/3(d3) -> stator flux/7(I_xs)
  MATLAB Function1/4(q3) -> stator flux/8(I_ys)
  stator flux/1(Lamda_ds) -> Real-Imag to Complex/1, Psi-alpha/1, Product1/1
  stator flux/2(Lamda_qs) -> Psi-beta/1, Real-Imag to Complex/2, Product/1
  Real-Imag to Complex/1 -> Complex to Magnitude-Angle/1

== system Conventional DTC/RTI Data/RTI Data Store/RTI Data Store ==
  RTI Data Store : Subsystem  mask(RTI_DATA_STORE){}
      mask help:
      | RTI Data Store Block. This block is used by RTI to store internal model dependent data. Deleting this block will result in data loss.
      |
      | NEVER DELETE, COPY, OR MODIFY THIS BLOCK!
      mask Help:
      | RTI Data Store Block. This block is used by RTI to store internal model dependent data. Deleting this block will result in data loss.
      | 
      | NEVER DELETE, COPY, OR MODIFY THIS BLOCK!
      mask Display: text(0.5, 0.5, ' ', 'HorizontalAlignment', 'center');

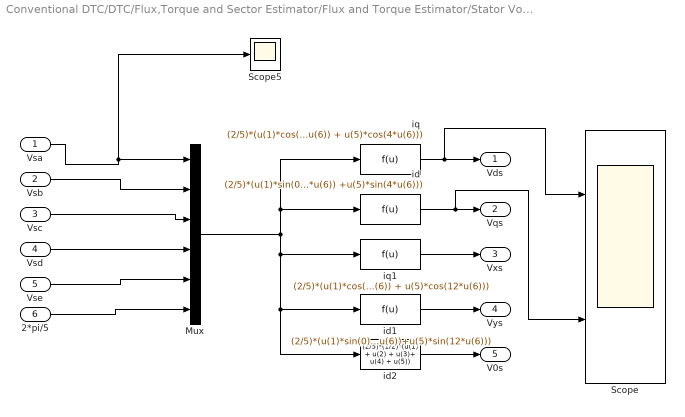
== system Conventional DTC/DTC/Flux,Torque and Sector Estimator/Flux and Torque Estimator/Stator Voltage  ==
  Vsa : Inport
  Vsb : Inport  Port=2
  Vsc : Inport  Port=3
  Vsd : Inport  Port=4
  Vse : Inport  Port=5
  2*pi/5 : Inport  Port=6
  Mux : Mux  Inputs=6
  Scope : Scope  NumInputPorts=2
  Scope5 : Scope
  id : Fcn  Expr=(2/5)*(u(1)*sin(0) + u(2)*sin(u(6)) +u(3)*sin(2*u(6)) +u(4)*sin(3*u(6)) +u(5)*sin(4*u(6)))
  id1 : Fcn  Expr=(2/5)*(u(1)*sin(0)+u(2)*sin(3*u(6))+u(3)*sin(6*u(6)) +u(4)*sin(9*u(6))+u(5)*sin(12*u(6)))
  id2 : Fcn  Expr=(2/5)*(1/2)*(u(1) + u(2) + u(3)+ u(4) + u(5))
  iq : Fcn  Expr=(2/5)*(u(1)*cos(0) + u(2)*cos(u(6)) + u(3)*cos(2*u(6)) + u(4)*cos(3*u(6)) + u(5)*cos(4*u(6)))
  iq1 : Fcn  Expr=(2/5)*(u(1)*cos(0) + u(2)*cos(3*u(6)) + u(3)*cos(6*u(6)) + u(4)*cos(9*u(6)) + u(5)*cos(12*u(6)))
  Vds : Outport
  Vqs : Outport  Port=2
  Vxs : Outport  Port=3
  Vys : Outport  Port=4
  V0s : Outport  Port=5
  wires:
  Vsd/1 -> Mux/4
  Vsc/1 -> Mux/3
  Vse/1 -> Mux/5
  Vsb/1 -> Mux/2
  Vsa/1 -> Scope5/1, Mux/1
  2*pi/5/1 -> Mux/6
  Mux/1 -> id2/1, id1/1, iq1/1, iq/1, id/1
  iq/1 -> Scope/1, Vds/1
  id/1 -> Scope/2, Vqs/1
  iq1/1 -> Vxs/1
  id1/1 -> Vys/1
  id2/1 -> V0s/1

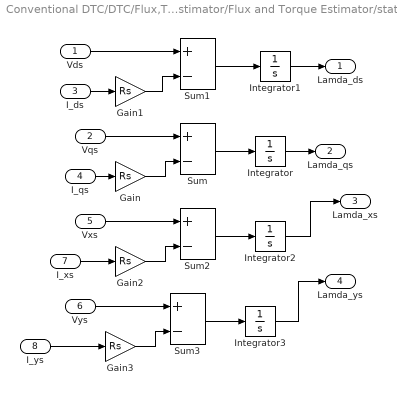
== system Conventional DTC/DTC/Flux,Torque and Sector Estimator/Flux and Torque Estimator/stator flux ==
  Vds : Inport
  Vqs : Inport  Port=2
  I_ds : Inport  Port=3
  I_qs : Inport  Port=4
  Vxs : Inport  Port=5
  Vys : Inport  Port=6
  I_xs : Inport  Port=7
  I_ys : Inport  Port=8
  Gain{,1..3} (4 alike) : Gain  Gain=Rs
  Integrator{,1..3} (4 alike) : Integrator
  Sum{,1..3} (4 alike) : Sum  Inputs=+-
  Lamda_ds : Outport
  Lamda_qs : Outport  Port=2
  Lamda_xs : Outport  Port=3
  Lamda_ys : Outport  Port=4
  wires:
  Vqs/1 -> Sum/1
  Gain/1 -> Sum/2
  Sum/1 -> Integrator/1
  Integrator/1 -> Lamda_qs/1
  Integrator1/1 -> Lamda_ds/1
  Sum1/1 -> Integrator1/1
  Gain1/1 -> Sum1/2
  Vds/1 -> Sum1/1
  I_qs/1 -> Gain/1
  I_ds/1 -> Gain1/1
  Vxs/1 -> Sum2/1
  Gain2/1 -> Sum2/2
  Sum2/1 -> Integrator2/1
  Integrator2/1 -> Lamda_xs/1
  I_xs/1 -> Gain2/1
  Vys/1 -> Sum3/1
  Gain3/1 -> Sum3/2
  Sum3/1 -> Integrator3/1
  Integrator3/1 -> Lamda_ys/1
  I_ys/1 -> Gain3/1

== system Conventional DTC/RTI Data/RTI Data Store/RTI Data Store/RTI Data Store ==
  RTI Data Store : Subsystem  mask(RTI_DATA_STORE){}
      mask help:
      | RTI Data Store Block. This block is used by RTI to store internal model dependent data. Deleting this block will result in data loss.
      |
      | NEVER DELETE, COPY, OR MODIFY THIS BLOCK!
      mask Help:
      | RTI Data Store Block. This block is used by RTI to store internal model dependent data. Deleting this block will result in data loss.
      | 
      | NEVER DELETE, COPY, OR MODIFY THIS BLOCK!
      mask Display: text(0.5, 0.5, ' ', 'HorizontalAlignment', 'center');

== system Conventional DTC/RTI Data/RTI Data Store/RTI Data Store/RTI Data Store/RTI Data Store ==

== matlab function Conventional DTC/DTC/switching table1/MATLAB Function ==
  data: sector input; v output; Hs input; Hmd input
function v=fcn(sector,Hs,Hmd)
v=1;
 if(sector==1)
    if(Hs==1 && Hmd==1)
        v=3;
    elseif(Hs==1 && Hmd==-1)
        v=9;
    elseif(Hs==-1 && Hmd==1)
        v=4;
    else
        v=8;
    end
 end
if(sector==2)
    if(Hs==1 && Hmd==1)
        v=4;
    elseif(Hs==1 && Hmd==-1)
        v=10;
    elseif(Hs==-1 && Hmd==1)
        v=5;
    else
        v=9;
    end
end
if(sector==3)
    if(Hs==1 && Hmd==1)
        v=5;
    elseif(Hs==1 && Hmd==-1)
        v=1;
    elseif(Hs==-1 && Hmd==1)
        v=6;
    else
        v=10;
    end
end
if(sector==4)
    if(Hs==1 && Hmd==1)
        v=6;
    elseif(Hs==1 && Hmd==-1)
        v=2;
    elseif(Hs==-1 && Hmd==1)
        v=7;
    else
        v=1;
    end
end
if(sector==5)
    if(Hs==1 && Hmd==1)
        v=7;
    elseif(Hs==1 && Hmd==-1)
        v=3;
    elseif(Hs==-1 && Hmd==1)
        v=8;
    else
        v=2;
    end
end
if(sector==6)
    if(Hs==1 && Hmd==1)
        v=8;
    elseif(Hs==1 && Hmd==-1)
        v=4;
    elseif(Hs==-1 && Hmd==1)
        v=9;
    else
        v=3;
    end
end
if(sector==7)
    if(Hs==1 && Hmd==1)
        v=9;
    elseif(Hs==1 && Hmd==-1)
        v=5;
    elseif(Hs==-1 && Hmd==1)
        v=10;
    else
        v=4;
    end
end
if(sector==8)
    if(Hs==1 && Hmd==1)
        v=10;
    elseif(Hs==1 && Hmd==-1)
        v=6;
    elseif(Hs==-1 && Hmd==1)
        v=1;
    else
        v=5;
    end
end
if(sector==9)
    if(Hs==1 && Hmd==1)
        v=1;
    elseif(Hs==1 && Hmd==-1)
        v=7;
    elseif(Hs==-1 && Hmd==1)
        v=2;
    else
        v=6;
    end
end
if(sector==10)
    if(Hs==1 && Hmd==1)
        v=2;
    elseif(Hs==1 && Hmd==-1)
        v=8;
    elseif(Hs==-1 && Hmd==1)
        v=3;
    else
        v=7;
    end
end
end

== matlab function Conventional DTC/DTC/switching table1/MATLAB Function1 ==
  data: v input; G output
function G  = fcn(v)
G=1;
if (v==1) || (v==11) ||(v==21) 
     G=1;
elseif(v==2) || (v==12) ||(v==22) 
     G=2;
elseif(v==3) || (v==13) ||(v==23) 
     G=3;
 elseif(v==4) ||(v==14) ||(v==24) 
     G=4;   
 elseif(v==5) || (v==15) ||(v==25) 
     G=5;   
elseif(v==6) || (v==16) ||(v==26) 
     G=6;
elseif(v==7) || (v==17) ||(v==27) 
     G=7;
elseif(v==8) || (v==18) ||(v==28) 
     G=8;
elseif(v==9) || (v==19) ||(v==29) 
     G=9;
elseif(v==10) || (v==20) ||(v==30) 
     G=10;
end

== matlab function Conventional DTC/DTC/switching table1/MATLAB Function2 ==
  data: G input; v output; S input
function v  = fcn(G,S)
v=1;
if (G==1)
  if (S==9) || (S==10) ||(S==1)  || (S==2) ||(S==3)
     v=1;
  elseif(S==4) || (S==5) ||(S==6)  || (S==7) ||(S==8)
     v=11;
  end
elseif (G==2)
  if (S==2) || (S==3) ||(S==4)  || (S==5) ||(S==6)
     v=2;
  elseif(S==7) || (S==8) ||(S==9)  || (S==10) ||(S==1)
     v=12;
  end
elseif (G==3)
  if (S==5) || (S==6) ||(S==7)  || (S==8) ||(S==9)
     v=3;
  elseif(S==10) || (S==1) ||(S==2)  || (S==3) ||(S==4)
     v=13;
  end
elseif (G==4)
  if (S==8) || (S==9) ||(S==10)  || (S==1) ||(S==2)
     v=4;
  elseif(S==3) || (S==4) ||(S==5)  || (S==6) ||(S==7)
     v=14;
  end
elseif (G==5)
  if (S==1) || (S==2) ||(S==3)  || (S==4) ||(S==5)
     v=5;
  elseif(S==6) || (S==7) ||(S==8)  || (S==9) ||(S==10)
     v=15;
  end  
elseif (G==6)
  if (S==4) || (S==5) ||(S==6)  || (S==7) ||(S==8)
     v=6;
  elseif(S==9) || (S==10) ||(S==1)  || (S==2) ||(S==3)
     v=16;
  end
elseif (G==7)
  if (S==7) || (S==8) ||(S==9)  || (S==10) ||(S==1)
     v=7;
  elseif(S==2) || (S==3) ||(S==4)  || (S==5) ||(S==6)
     v=17;
  end
elseif (G==8)
  if (S==10) || (S==1) ||(S==2)  || (S==3) ||(S==4)
     v=8;
  elseif (S==5) ||(S==6)  || (S==7) ||(S==8)|| (S==9)
     v=18;
  end
elseif (G==9)
  if (S==3) || (S==4) ||(S==5)  || (S==6) ||(S==7)
     v=9;
  elseif(S==8) || (S==9) ||(S==10)  || (S==1) ||(S==2)
     v=19;
  end  
elseif (G==10)
  if (S==6) || (S==7) ||(S==8)  || (S==9) ||(S==10)
     v=10;
  elseif(S==1) || (S==2) || (S==3) ||(S==4)  || (S==5)
     v=20;
  end
end

== matlab function Conventional DTC/DTC/Flux,Torque and Sector Estimator/MATLAB Function2 ==
  data: theta input; sector output
function sector =SECTOR(theta)
if(theta>-pi/10 && theta<=pi/10)
    sector=1;
elseif(theta>pi/10 && theta<=3*pi/10)
    sector=2;
elseif(theta>3*pi/10 && theta<=pi/2)
    sector=3;
elseif(theta>pi/2 && theta<=7*pi/10)
    sector=4;
elseif(theta>7*pi/10 && theta<=9*pi/10)
    sector=5;
elseif(theta>-9*pi/10 && theta<=-7*pi/10)
    sector=7;
elseif(theta>-7*pi/10 && theta<=-pi/2)
    sector=8;
elseif(theta>-pi/2 && theta<=-3*pi/10)
    sector=9;
elseif(theta>-3*pi/10 && theta<=-pi/10)
    sector=10;        
else
    sector=6;
end

== matlab function Conventional DTC/DTC/Flux,Torque and Sector Estimator/Flux and Torque Estimator/MATLAB Function1 ==
  data: a input; d1 output; b input; c input; d input; e input; th input; q1 output; d3 output; q3 output
function [d1,q1,d3,q3]= fcn(a,b,c,d,e,th)
d1=(2/5)*(a+(b*cos(th))+(c*cos(2*th))+(d*cos(3*th))+(e*cos(4*th)));
q1=(2/5)*(((b*sin(th))+(c*sin(2*th))+(d*sin(3*th))+(e*sin(4*th))));
d3=(2/5)*(a+(b*cos(3*th))+(c*cos(6*th))+(d*cos(9*th))+(e*cos(12*th)));
q3=(2/5)*(((b*sin(3*th))+(c*sin(6*th))+(d*sin(9*th))+(e*sin(12*th))));
end

== matlab function Conventional DTC/DTC/Flux,Torque and Sector Estimator/MATLAB Function1 ==
  data: theta input; sector output
function sector =SECTOR(theta)
if(theta>-pi/10 && theta<=pi/10)
    sector=1;
elseif(theta>pi/10 && theta<=3*pi/10)
    sector=2;
elseif(theta>3*pi/10 && theta<=pi/2)
    sector=3;
elseif(theta>pi/2 && theta<=7*pi/10)
    sector=4;
elseif(theta>7*pi/10 && theta<=9*pi/10)
    sector=5;
elseif(theta>-9*pi/10 && theta<=-7*pi/10)
    sector=7;
elseif(theta>-7*pi/10 && theta<=-pi/2)
    sector=8;
elseif(theta>-pi/2 && theta<=-3*pi/10)
    sector=9;
elseif(theta>-3*pi/10 && theta<=-pi/10)
    sector=10;        
else
    sector=6;
end

== matlab function Conventional DTC/Phase Voltages/MATLAB Function1 ==
  data: Sa input; vas output; Sb input; Sc input; Sd input; Se input; Vdc input; vbs output; vcs output; vds output; ves output
function [vas,vbs,vcs,vds,ves] = fcn(Sa,Sb,Sc,Sd,Se,Vdc)
vas=(Vdc/5)*(4*Sa-Sb-Sc-Sd-Se);
vbs=(Vdc/5)*(-Sa+4*Sb-Sc-Sd-Se);
vcs=(Vdc/5)*(-Sa-Sb+4*Sc-Sd-Se);
vds=(Vdc/5)*(-Sa-Sb-Sc+4*Sd-Se);
ves=(Vdc/5)*(-Sa-Sb-Sc-Sd+4*Se);

== matlab function Conventional DTC/DTC/Control Pulses ==
  data: v input; sa output; sb output; sc output; sd output; se output
function [sa,sb,sc,sd,se]= fcn(v)
%#codegen
sa=1;
sb=1;
sc=0;
sd=0;
se=1;
if(v==1)
    sa=1;
    sb=1;
    sc=0;
    sd=0;
    se=1;
end
if(v==2)
    sa=1;
    sb=1;
    sc=0;
    sd=0;
    se=0;
end
if(v==3)
    sa=1;
    sb=1;
    sc=1;
    sd=0;
    se=0;
end
if(v==4)
    sa=0;
    sb=1;
    sc=1;
    sd=0;
    se=0;
end
if(v==5)
    sa=0;
    sb=1;
    sc=1;
    sd=1;
    se=0;
end
if(v==6)
    sa=0;
    sb=0;
    sc=1;
    sd=1;
    se=0;
end
if(v==7)
    sa=0;
    sb=0;
    sc=1;
    sd=1;
    se=1;
end
if(v==8)
    sa=0;
    sb=0;
    sc=0;
    sd=1;
    se=1;
end
if(v==9)
    sa=1;
    sb=0;
    sc=0;
    sd=1;
    se=1;
end
if(v==10)
    sa=1;
    sb=0;
    sc=0;
    sd=0;
    se=1;
end
if(v==11)
    sa=1;
    sb=0;
    sc=0;
    sd=0;
    se=0;
end
if(v==12)
    sa=1;
    sb=1;
    sc=1;
    sd=0;
    se=1;
end
if(v==13)
    sa=0;
    sb=1;
    sc=0;
    sd=0;
    se=0;
end
if(v==14)
    sa=1;
    sb=1;
    sc=1;
    sd=1;
    se=0;
end
if(v==15)
    sa=0;
    sb=0;
    sc=1;
    sd=0;
    se=0;
end
if(v==16)
    sa=0;
    sb=1;
    sc=1;
    sd=1;
    se=1;
end
if(v==17)
    sa=0;
    sb=0;
    sc=0;
    sd=1;
    se=0;
end
if(v==18)
    sa=1;
    sb=0;
    sc=1;
    sd=1;
    se=1;
end
if(v==19)
    sa=0;
    sb=0;
    sc=0;
    sd=0;
    se=1;
end
if(v==20)
    sa=1;
    sb=1;
    sc=0;
    sd=1;
    se=1;
end
if(v==21)
    sa=0;
    sb=1;
    sc=0;
    sd=0;
    se=1;
end
if(v==22)
    sa=1;
    sb=1;
    sc=0;
    sd=1;
    se=0;
end
if(v==23)
    sa=1;
    sb=0;
    sc=1;
    sd=0;
    se=0;
end
if(v==24)
    sa=0;
    sb=1;
    sc=1;
    sd=0;
    se=1;
end
if(v==25)
    sa=0;
    sb=1;
    sc=0;
    sd=1;
    se=0;
end
if(v==26)
    sa=1;
    sb=0;
    sc=1;
    sd=1;
    se=0;
end
if(v==27)
    sa=0;
    sb=0;
    sc=1;
    sd=0;
    se=1;
end
if(v==28)
    sa=0;
    sb=1;
    sc=0;
    sd=1;
    se=1;
end
if(v==29)
    sa=1;
    sb=0;
    sc=0;
    sd=1;
    se=0;
end
if(v==30)
    sa=1;
    sb=0;
    sc=1;
    sd=0;
    se=1;
end
